simulink model "Speed_Control_of_BLDC_Motor_with_PWM"  (R2025a)
settings: Solver=ode45  StartTime=0.0  StopTime=13  RelTol=1e-3  EnableMultiTasking=on
undefined symbols (not defined in the file): Ion, Lithium
libraries: spsMosfetLib x6, spsBatteryLib x1, spsCurrentMeasurementLib x1, simulink x1, spsMeanLib x1, slpidlib x1, spsPWMGeneratorDCDCLib x1, spsPermanentMagnetSynchronousMachineLib x1, spspowerguiLib x1
settings Model: Creator=Aslam  LastModifiedBy=Laptop
settings SolverCC: AlgebraicLoopSolver=TrustRegion
settings DataIOCC: LimitDataPoints=on  SaveFormat=Array  ReturnWorkspaceOutputs=off
settings OptimizationCC: LifeSpan=inf
settings DebuggingCC: SolverPrmCheckMsg=warning  UnconnectedInputMsg=warning  UnconnectedOutputMsg=warning  UnconnectedLineMsg=warning  SFUnexpectedBacktrackingDiag=warning  SFNoUnconditionalDefaultTransitionDiag=warning  SFExecutionAtInitializationDiag=none  ArithmeticOperatorsInVariantConditions=warning
settings HardwareCC: ProdBitPerPointer=32.0  ProdBitPerSizeT=32.0  ProdBitPerPtrDiffT=32.0  ProdLargestAtomicFloat=None  ProdIntDivRoundTo=Undefined  ProdEndianess=Unspecified  ProdWordSize=32.0  ProdHWDeviceType=32-bit Generic
settings ModelReferenceCC: EnableRefExpFcnMdlSchedulingChecks=on  PropagateSignalLabelsOutOfModel=off
settings SFSimCC: SimUseLocalCustomCode=off  CustomCodeUndefinedFunction=UseInterfaceOnly
settings RTWCC: RTWUseLocalCustomCode=off  GPUComputeCapability=3.5
settings CodeAppCC: StateflowObjectComments=on
settings GRTTargetCC: TargetLangStandard=C89/C90 (ANSI)
settings ConfigComp: CovMetricSettings=dw  CovSaveCumulativeToWorkspaceVar=on  CovSaveSingleToWorkspaceVar=on  CovExternalEMLEnable=off  CovSFcnEnable=off
settings SimscapeCC: SimscapeNormalizeSystem=off

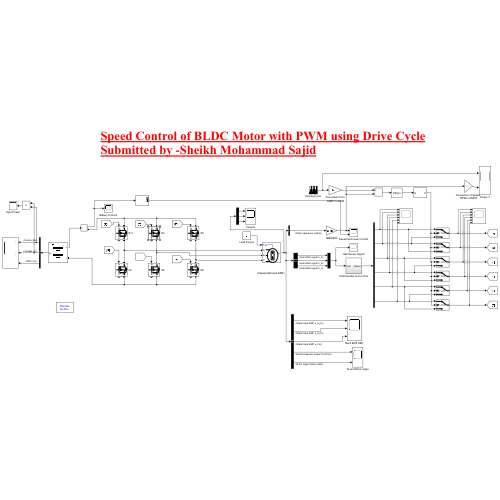
[thumbnail: Simulink's stored preview of the top-level diagram]
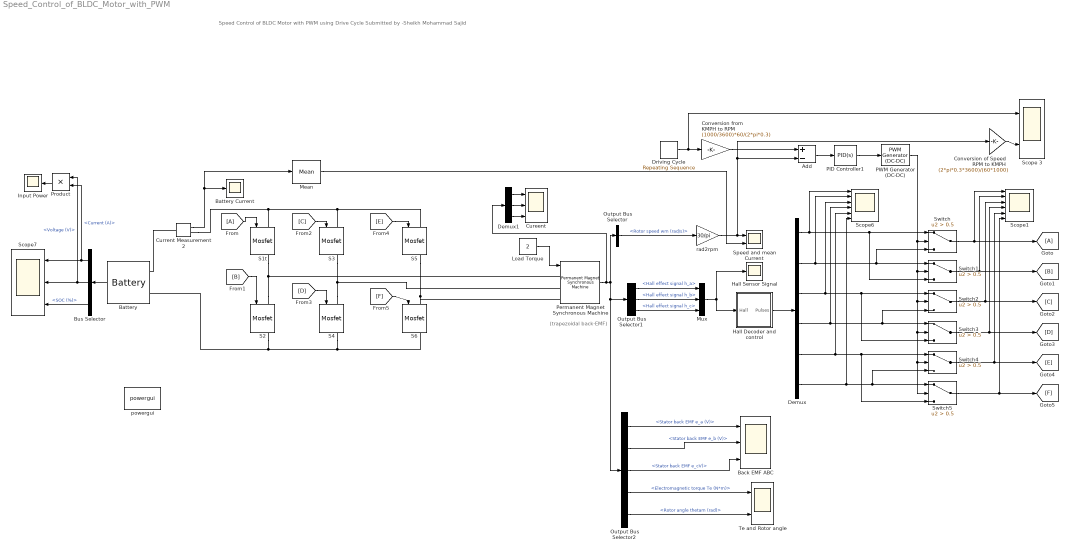
== system Speed_Control_of_BLDC_Motor_with_PWM ==
  note: Speed Control of BLDC Motor with PWM using Drive Cycle
      | Submitted by -Sheikh Mohammad Sajid
  note: (trapezoidal back-EMF)
  Add : Sum  Inputs=+-
  Back EMF ABC : Scope  NumInputPorts=3
      settings: ActiveDisplayYMinimum=-18.332  ActiveDisplayYMaximum=18.33178
  Battery : spsBatteryLib/Battery  BatType=Lithium-Ion  NomV=48  NomQ=6.5  SOC=80  Batt_Tr=30  PresetModel=on  MaxQ=6.5  MinV=36  FullV=55.8714  Dis_rate=2.8261  R=0.073846  Normal_OP=5.8783  expZone="[51.8585     0.319348]"
      settings: LibrarySourceBlock=electricdrivelib/Extra Sources/Battery
  Battery Current : Scope
      settings: ActiveDisplayYMinimum=-1.14222  ActiveDisplayYMaximum=1.12492  DataLoggingVariableName=ScopeData2  DataLoggingSaveFormat=Array
  Bus Selector : BusSelector  OutputSignals=Current (A),Voltage (V),SOC (%)
  "Conversion from KMPH to RPM " : Gain  Gain=(1000/3600)*60/(2*pi*0.3)
  Conversion of Speed RPM to KMPH : Gain  Gain=(2*pi*0.3*3600)/(60*1000)  SaturateOnIntegerOverflow=on  OutDataTypeStr=Inherit: Same as input  ParamDataTypeStr=Inherit: Same as input
  Cureent : Scope  NumInputPorts=3
      settings: ActiveDisplayYMinimum=-5.8817  ActiveDisplayYMaximum=7.86163  DataLoggingVariableName=ScopeData3
  Current Measurement2 : spsCurrentMeasurementLib/Current Measurement  PhasorSimulation=off  OutputType=Complex  PSBequivalent=0
  Demux : Demux  Outputs=6
  Demux1 : Demux  Outputs=3
  Driving Cycle : simulink/Sources/Repeating Sequence  rep_seq_t=[0 1 2 3 4 5 6 7 8 9 10 11 11.0001 12 13]  rep_seq_y=[0 0 10 10 0 0 20 20 0 0 35 35 25 25 0]
  From : From
  Goto : Goto
  Hall Decoder and control : Subsystem
  Hall Sensor Signal : Scope
      settings: DataLoggingVariableName=ScopeData4  DataLoggingSaveFormat=Array
  Input Power : Scope
      settings: ActiveDisplayYMinimum=-4694.35057  ActiveDisplayYMaximum=3211.96925  DataLoggingVariableName=ScopeData5
  Load Torque : Constant  Value=2
  Mean : spsMeanLib/Mean  Freq=50  Vinit=0  Ts=0
  Mux : Mux  Inputs=3
  Output Bus Selector : BusSelector  OutputSignals=Rotor speed wm (rad/s)
  Output Bus Selector1 : BusSelector  OutputSignals=Hall effect signal h_a,Hall effect signal h_b,Hall effect signal h_c
  Output Bus Selector2 : BusSelector  OutputSignals=Stator back EMF e_a (V),Stator back EMF e_b (V),Stator back EMF e_cV),Electromagnetic torque Te (N*m),Rotor angle thetam (rad)
  PID Controller1 : slpidlib/PID Controller  Controller=PID  Form=Parallel  TimeDomain=Continuous-time  UseExternalTs=off  SampleTime=-1  IntegratorMethod=Forward Euler  FilterMethod=Forward Euler  ControllerParametersSource=internal  P=1  I=1  UseKiTs=off  D=0  UseExternalDerivativeSource=off  N=100  UseFilter=on  TunerSelectOption=Transfer Function Based (PID Tuner App)  InitialConditionSource=internal  InitialConditionForIntegrator=0  InitialConditionForFilter=0  DifferentiatorICPrevScaledInput=0  ExternalReset=none  TrackingMode=off  Kt=1  LimitOutput=off  SatLimitsSource=internal  UpperSaturationLimit=inf  LowerSaturationLimit=-inf  LinearizeAsGain=on  AntiWindupMode=none  Kb=1  LimitIntegrator=off  UpperIntegratorSaturationLimit=inf  LowerIntegratorSaturationLimit=-inf  POutMin=[]  POutMax=[]  IOutMin=[]  IOutMax=[]  DOutMin=[]  DOutMax=[]  NOutMin=[]  NOutMax=[]  SumOutMin=[]  SumOutMax=[]  SaturationOutMin=[]  SaturationOutMax=[]  PParamMin=[]  PParamMax=[]  IParamMin=[]  IParamMax=[]  DParamMin=[]  DParamMax=[]  NParamMin=[]  NParamMax=[]  KbParamMin=[]  KbParamMax=[]  KtParamMin=[]  KtParamMax=[]  KbOutMin=[]  KbOutMax=[]  KtOutMin=[]  KtOutMax=[]  IntegratorOutMin=[]  IntegratorOutMax=[]  FilterOutMin=[]  FilterOutMax=[]  SumI1OutMin=[]  SumI1OutMax=[]  SumI2OutMin=[]  SumI2OutMax=[]  SumI3OutMin=[]  SumI3OutMax=[]  SumI4OutMin=[]  SumI4OutMax=[]  SumDOutMin=[]  SumDOutMax=[]  DifferentiatorOutMin=[]  DifferentiatorOutMax=[]  FilterDiffOutCoefMin=[]  FilterDiffOutCoefMax=[]  ReciprocalOutMin=[]  ReciprocalOutMax=[]  SumDenOutMin=[]  SumDenOutMax=[]  SumNumOutMin=[]  SumNumOutMax=[]  DivideOutMin=[]  DivideOutMax=[]  UdiffTsProdOutMin=[]  UdiffTsProdOutMax=[]  NTsProdOutMin=[]  NTsProdOutMax=[]  UintegralTsProdOutMin=[]  UintegralTsProdOutMax=[]  UngainTsProdOutMin=[]  UngainTsProdOutMax=[]  ClampingZeroOutDataTypeStr=Inherit: Inherit via back propagation  ClampingZeroOutMin=[]  ClampingZeroOutMax=[]  FilterDenConstantOutDataTypeStr=Inherit: Inherit via back propagation  FilterDenConstantOutMin=[]  FilterDenConstantOutMax=[]  PCopyOutDataTypeStr=Inherit: Inherit via back propagation  PCopyOutMin=[]  PCopyOutMax=[]  NCopyOutDataTypeStr=Inherit: Inherit via back propagation  NCopyOutMin=[]  NCopyOutMax=[]  IntegratorContinuousStateAttributes=''  IntegratorStateMustResolveToSignalObject=off  IntegratorRTWStateStorageClass=Auto  FilterContinuousStateAttributes=''  FilterStateMustResolveToSignalObject=off  FilterRTWStateStorageClass=Auto  ParallelPVariant=InternalParameters  IdealPVariant=Disabled  IVariant=InternalParameters  DVariant=InternalParameters  IntegratorVariant=Continuous  SatVariant=Disabled  AWVariant=Passthrough  PCopyVariant=Disabled  TRVariant=Disabled  FdbkBlocksVariant=Forward  IdealPFdbkVariant=Disabled  SatFdbkVariant=Disabled  DerivativeFilterVariant=ContFilter  NVariant=InternalParameters  NCopyVariant=Disabled  FilterICVariant=InternalICsFilter  IntegratorICVariant=InternalICs  ExternalResetVariant=Disabled  TRSumVariant=Passthrough  SumFdbkVariant=Disabled  SumVariant=Sum_PID  TsampFilterVariant=InternalTs  TsampNgainVariant=Passthrough  TsampIntegralVariant=Disabled_SignalSpec  ExternalSaturationOutDataTypeStr=Inherit: Same as second input  DerivativeSourceVariant=ErrorSignal  PreIntVariant=InternalPreInt
  PWM Generator (DC-DC) : spsPWMGeneratorDCDCLib/PWM Generator (DC-DC)  Fsw=5000  Ts=0
  Permanent Magnet Synchronous Machine : spsPermanentMagnetSynchronousMachineLib/Permanent Magnet Synchronous Machine  NbPhases=3  FluxDistribution=Trapezoidal  RotorType=Round  MechanicalLoad=Torque Tm  PresetModel=No  ShowDetailedParameters=on  MeasurementBus=off  Resistance=0.2  Inductance=8.5e-3  dqInductances=[8.5e-3,8.5e-3]  La=0.000835  MachineConstant=Flux linkage established by magnets (V.s)  Flux=0.175  VoltageCst=146.6077  TorqueCst=1.4  Flat=120  Mechanical=[0.12,0.005,4]  PolePairs=4  InitialConditions=[0,0,0,0]  InitialConditions5ph=[0 0 0 0 0 0]  RefAngle=90 degrees behind phase A axis (modified Park)  IterativeDiscreteModel=Trapezoidal non iterative  TsBlock=-1  TsPowergui=0
  Product : Product
  S1t : spsMosfetLib/Mosfet  Ron=0.1  Lon=0  Rd=0.01  Vfd=0  IC=0  Rs=1e5  Cs=inf  Measurements=on
  S{2..6} (5 alike) : spsMosfetLib/Mosfet  Ron=0.1  Lon=0  Rd=0.01  Vfd=0  IC=0  Rs=1e5  Cs=inf  Measurements=on
  Scope 3 : Scope  NumInputPorts=2
      settings: Title=Driving Cycle Speed in KMPH  ActiveDisplayYMinimum=-1.25  ActiveDisplayYMaximum=11.25
  Scope1 : Scope  NumInputPorts=6
      settings: Title=Switching Pulse to S1  ActiveDisplayYMinimum=-0.125  ActiveDisplayYMaximum=1.125
  Scope6 : Scope  NumInputPorts=6
      settings: ActiveDisplayYMinimum=-0.125  ActiveDisplayYMaximum=1.125  DataLoggingVariableName=ScopeData8
  Scope7 : Scope  NumInputPorts=3
      settings: Title=Battery Current in amps  ActiveDisplayYMinimum=-83.35071  ActiveDisplayYMaximum=65.06304  DataLoggingVariableName=ScopeData9
  Speed and mean Current : Scope  NumInputPorts=2
      settings: ActiveDisplayYMinimum=-39.82461  ActiveDisplayYMaximum=348.41434  DataLoggingVariableName=ScopeData10
  Switch{,1..5} (6 alike) : Switch  Criteria=u2 > Threshold  Threshold=0.5  SaturateOnIntegerOverflow=off  InputSameDT=off
  Te and Rotor angle : Scope  NumInputPorts=2
      settings: ActiveDisplayYMinimum=-83.47582  ActiveDisplayYMaximum=45.89727
  powergui : spspowerguiLib/powergui  Priority=1  SimulationMode=Discrete  SampleTime=5e-6  frequency=60  Iterations=50  frequencyindice=0  Pbase=100e6  ErrMax=1e-4  UnitsV=kV  UnitsW=MW  buscounter=0  FunctionMessages=off  echomessages=off  EnableUseOfTLC=off  CurrentSourceSwitches=off  DisableSnubberDevices=off  DisableRonSwitches=off  DisableVfSwitches=off  DisplayEquations=off  AutomaticDiscreteSolvers=off  SolverType=Tustin  Interpol=off  ExternalGateDelay=off  methode=off  Ts=0  x0status=blocks  SPID=off  SwTol=0  HookPort=off  NonlinearTolerance=1e-4  nMaxIteration=100  ContinueOnMaxIteration=off  RestoreLinks=warning  ResistiveCurrentMeasurement=off  Frange=[0:2:500]  Ylog=off  Xlog=on  ShowGrid=off  save=off  variable=ZData  structure=0  ZoomFFT=off  StartTime=0.0  cycles=1  DisplayStyle=1  fundamental=60  FreqAxis=off  MaxFrequency=1000  frequencyindicesteady=1  RmsSteady=1  display=off
  rad2rpm : Gain  Gain=30/pi  SaturateOnIntegerOverflow=on  OutDataTypeStr=Inherit: Same as input  ParamDataTypeStr=Inherit: Same as input
  wires:
  Load Torque/1 -> Permanent Magnet Synchronous Machine/1
  Output Bus Selector/1 -> rad2rpm/1  "<Rotor speed wm (rad/s)>"
  rad2rpm/1 -> Conversion of Speed RPM to KMPH/1, Add/2, Speed and mean Current/1
  Output Bus Selector1/1 -> Mux/1  "<Hall effect signal h_a>"
  Output Bus Selector1/2 -> Mux/2  "<Hall effect signal h_b>"
  Output Bus Selector1/3 -> Mux/3  "<Hall effect signal h_c>"
  Mux/1 -> Hall Decoder and control/1("Hall "), Hall Sensor Signal/1
  Hall Decoder and control/1(Pulses) -> Demux/1
  Current Measurement2/1 -> Mean/1, Battery Current/1
  From/1 -> S1t/1
  [B] -> S2/1
  [C] -> S3/1
  [D] -> S4/1
  [E] -> S5/1
  [F] -> S6/1
  Demux/4 -> Switch2/3, Switch3/1, Scope6/4
  Mean/1 -> Speed and mean Current/2
  Battery/1 -> Bus Selector/1
  Bus Selector/1 -> Scope7/1, Product/2  "<Current (A)>"
  Bus Selector/2 -> Product/1, Scope7/2  "<Voltage (V)>"
  Bus Selector/3 -> Scope7/3  "<SOC (%)>"
  Output Bus Selector2/1 -> Back EMF ABC/1  "<Stator back EMF e_a (V)>"
  Output Bus Selector2/2 -> Back EMF ABC/2  "<Stator back EMF e_b (V)>"
  Output Bus Selector2/3 -> Back EMF ABC/3  "<Stator back EMF e_cV)>"
  Output Bus Selector2/4 -> Te and Rotor angle/1  "<Electromagnetic torque Te (N*m)>"
  Output Bus Selector2/5 -> Te and Rotor angle/2  "<Rotor angle thetam (rad)>"
  Product/1 -> Input Power/1
  Permanent Magnet Synchronous Machine/1 -> Demux1/1, Output Bus Selector/1, Output Bus Selector2/1, Output Bus Selector1/1
  Demux1/1 -> Cureent/1
  Demux1/2 -> Cureent/2
  Demux1/3 -> Cureent/3
  Demux/5 -> Switch5/3, Switch4/1, Scope6/5
  Demux/6 -> Switch4/3, Switch5/1, Scope6/6
  Demux/3 -> Switch3/3, Switch2/1, Scope6/3
  Demux/1 -> Switch1/3, Switch/1, Scope6/1
  Demux/2 -> Switch/3, Switch1/1, Scope6/2
  Switch5/1 -> Scope1/6, [F]
  Switch4/1 -> Scope1/5, [E]
  Switch3/1 -> Scope1/4, [D]
  Switch2/1 -> Scope1/3, [C]
  Switch1/1 -> Scope1/2, [B]
  Switch/1 -> Scope1/1, Goto/1
  Add/1 -> PID Controller1/1
  "Conversion from KMPH to RPM "/1 -> Add/1
  PID Controller1/1 -> PWM Generator (DC-DC)/1
  PWM Generator (DC-DC)/1 -> Switch5/2, Switch4/2, Switch3/2, Switch2/2, Switch1/2, Switch/2
  Driving Cycle/1 -> Scope 3/1, "Conversion from KMPH to RPM "/1
  Conversion of Speed RPM to KMPH/1 -> Scope 3/2
  connections:
  Current Measurement2/RConn1 -- S1t/LConn1 -- S3/LConn1 -- S5/LConn1
  S2/RConn1 -- S4/RConn1 -- S6/RConn1 -- Battery/LConn2
  S4/LConn1 -- Permanent Magnet Synchronous Machine/LConn2 -- S3/RConn1
  S6/LConn1 -- Permanent Magnet Synchronous Machine/LConn3 -- S5/RConn1
  S2/LConn1 -- S1t/RConn1 -- Permanent Magnet Synchronous Machine/LConn1
  Current Measurement2/LConn1 -- Battery/LConn1

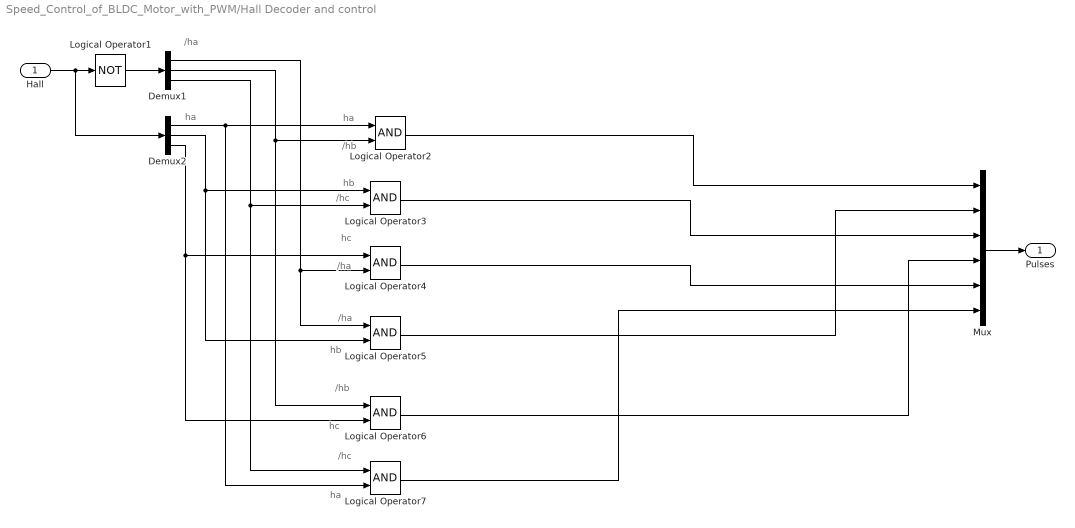
== system Speed_Control_of_BLDC_Motor_with_PWM/Hall Decoder and control ==
  note: ha
  note: /hc
  note: hc
  note: /hb
  note: hb
  note: /ha
  note: /ha
  note: hc
  note: /hc
  note: hb
  note: /hb
  note: ha
  note: ha
  note: /ha
  "Hall " : Inport
  Demux1 : Demux  Outputs=3
  Demux2 : Demux  Outputs=3
  Logical Operator1 : Logic  Operator=NOT  AllPortsSameDT=off  OutDataTypeStr=boolean
  Logical Operator{2..7} (6 alike) : Logic  AllPortsSameDT=off  OutDataTypeStr=boolean
  Mux : Mux  Inputs=6
  Pulses : Outport
  wires:
  Demux1/3 -> Logical Operator7/1, Logical Operator3/2
  "Hall "/1 -> Demux2/1, Logical Operator1/1
  Demux1/1 -> Logical Operator5/1, Logical Operator4/2
  Demux2/1 -> Logical Operator7/2, Logical Operator2/1
  Demux1/2 -> Logical Operator6/1, Logical Operator2/2
  Demux2/2 -> Logical Operator5/2, Logical Operator3/1
  Logical Operator1/1 -> Demux1/1
  Demux2/3 -> Logical Operator6/2, Logical Operator4/1
  Mux/1 -> Pulses/1
  Logical Operator2/1 -> Mux/1
  Logical Operator3/1 -> Mux/3
  Logical Operator4/1 -> Mux/5
  Logical Operator5/1 -> Mux/2
  Logical Operator6/1 -> Mux/4
  Logical Operator7/1 -> Mux/6
